simulink model "GIM81115_6_motor_model_prev_verision"  (R2024a)
settings: Solver=FixedStepAuto  StartTime=0.0  StopTime=inf  RelTol=1e-3
undefined symbols (not defined in the file): HS, IO291
libraries: speedgoatlib_IO691 x9, canmsglib x8, aru_toolbox x1, speedgoatlib_IO291 x1
settings Model: SimulationMode=external  ExtModeEnableFloating=off  Creator=claro  LastModifiedBy=user
settings SolverCC: ConcurrentTasks=on  PositivePriorityOrder=on
settings OptimizationCC: BlockReduction=off  OptimizeBlockIOStorage=off
settings DebuggingCC: TasksWithSamePriorityMsg=none
settings HardwareCC: ProdBitPerLong=64  ProdLongLongMode=on  ProdHWDeviceType=Intel->x86-64 (Linux 64)
settings RTWCC: Description=Speedgoat Real-Time Target Machine  SystemTargetFile=speedgoat.tlc  TemplateMakefile=slrealtime_default_tmf  Toolchain=Simulink Real-Time Toolchain  BuildConfiguration=Faster Runs  CodeExecutionProfiling=on  TargetLang=C++
settings SimulinkRealTimeTargetCC: InstructionSetFMA=off  LogToMDFFile=off

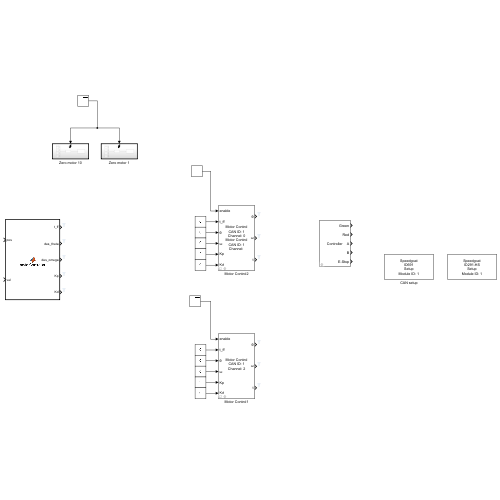
[thumbnail: Simulink's stored preview of the top-level diagram]
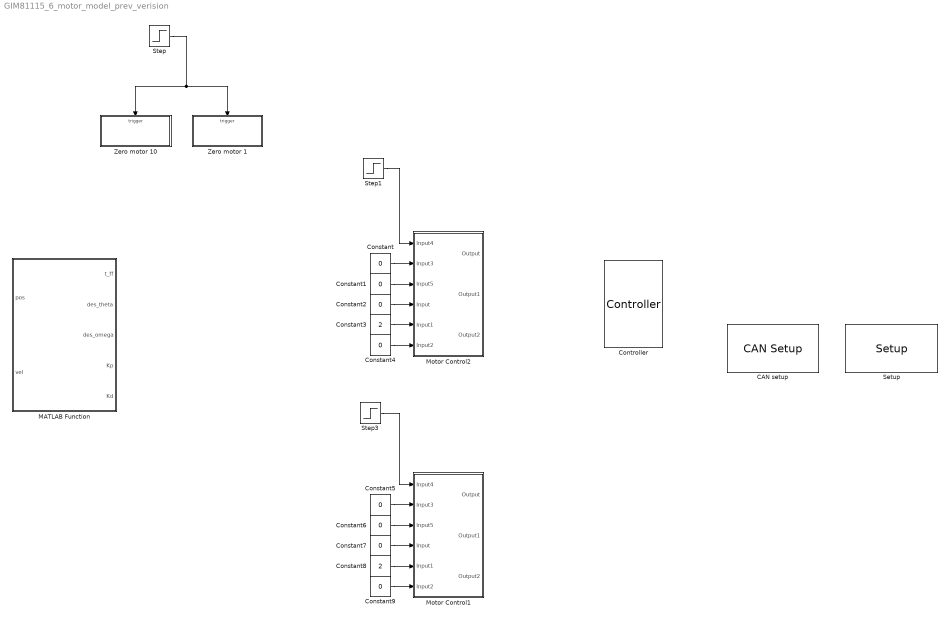
== system GIM81115_6_motor_model_prev_verision ==
  CAN setup : speedgoatlib_IO691/Legacy/CAN Setup   moduletype=IO691  id=1  pciSlot=-1  chn1=CAN (HS)  chn2=CAN (HS)  chn3=Disabled  chn4=Disabled  initStruct=[]  termStruct=[struct('Channel',1,'Protocol','CAN','BRS',0,'Type','Standard','Identifier',1,'Data',[255, 255, 255, 255, 255, 255, 255, 253],'Pause',0.001), struct('Channel',2,'Protocol','CAN','BRS',0,'Type','Standard','Identifier',2,'Data',[255, 255, 255, 255, 255, 255, 255, 253],'Pause',0.001)]  ArbitrationbdrChn1=1.0 MBaud  ArbitrationManbdrChn1=[2,8,31,8]  FdbdrChn1=1.0 MBaud  FdManbdrChn1=[2,8,31,8]  ArbitrationbdrChn2=1.0 MBaud  ArbitrationManbdrChn2=[2,8,31,8]  FdbdrChn2=1.0 MBaud  FdManbdrChn2=[2,8,31,8]  ArbitrationbdrChn3=1.0 MBaud  ArbitrationManbdrChn3=[2,8,31,8]  FdbdrChn3=5.0 MBaud  FdManbdrChn3=[2,2,5,2]  ArbitrationbdrChn4=1.0 MBaud  ArbitrationManbdrChn4=[2,8,31,8]  FdbdrChn4=5.0 MBaud  FdManbdrChn4=[2,2,5,2]  moduleInitValues=[691 1 -1 -1]
      settings: SourceProductName=IO691
  Constant{,1..2,4..7,9} (8 alike) : Constant  Value=0
  Constant3 : Constant  Value=2
  Constant8 : Constant  Value=2
  Controller : aru_toolbox/Controller
      settings: SourceProductName=ARU Toolbox
  MATLAB Function : MATLAB Function  TreatAsAtomicUnit=on
  Motor Control1 : Subsystem  AncestorBlock=aru_toolbox/Motor Control  mask(Motor Control){id=1, channel=2, offset=0}
      mask prompts: offset "Position Offset (rad)"
      mask help: Generic control block for motors running Ben Katz's motor control firmware. (https://github.com/bgkatz/motorcontrol)
      mask init:
      | % set_param([gcb '/write/CAN pack'],'MsgIdentifier',sprintf('%d',id));
      | set_param([gcb '/write/CAN Write Command'],'channel',sprintf('%d',channel));
      | set_param([gcb '/read/CAN Read State'],'channel',sprintf('%d',channel));
      | 
      | % set_param([gcb '/enable/CAN pack'],'MsgIdentifier',sprintf('%d',id));
      | set_param([gcb '/enable/CAN Write Motor Mode'],'channel',sprintf('%d',channel));
      | % motor termination message
      | % set_param([gcb '/CAN setup'],'termStruct',sprintf("[struct('Channel',%d,'Protocol','CAN','BRS',0,'Type','Standard','Identifier',%d,'Data',[255, 255, 255, 255, 255, 255, 255, 253],'Pause',0.001)]", channel, id))
      mask TypeOptions channel: 1 | 2
      mask DialogControl ParameterGroupVar Prompt: CAN
      mask DialogControl Container4 Prompt: Control
      mask Display:
      | fprintf('Motor Control\nCAN ID: %c\nChannel: %c\n', get_param(gcb,'id'), get_param(gcb,'channel'));
      | port_label('input',1,'enable');
      | port_label('input',2,'t_ff');
      | port_label('input',3,'θ');
      | port_label('input',4,'ω');
      | port_label('input',5,'Kp');
      | port_label('input',6,'Kd');
      | port_label('output',1,'θ');
      | port_label('output',2,'ω');
      | port_label('output',3,'t');
  Motor Control2 : Subsystem  AncestorBlock=aru_toolbox/Motor Control  mask(Motor Control){id=10, channel=1, offset=0}
      mask prompts: offset "Position Offset (rad)"
      mask help: Generic control block for motors running Ben Katz's motor control firmware. (https://github.com/bgkatz/motorcontrol)
      mask init: same as GIM81115_6_motor_model_prev_verision/Motor Control1
      mask TypeOptions channel: 1 | 2
      mask DialogControl ParameterGroupVar Prompt: CAN
      mask DialogControl Container4 Prompt: Control
      mask Display:
      | fprintf('Motor Control\nCAN ID: %c\nChannel: %c\n', get_param(gcb,'id'), get_param(gcb,'channel'));
      | port_label('input',1,'enable');
      | port_label('input',2,'t_ff');
      | port_label('input',3,'θ');
      | port_label('input',4,'ω');
      | port_label('input',5,'Kp');
      | port_label('input',6,'Kd');
      | port_label('output',1,'θ');
      | port_label('output',2,'ω');
      | port_label('output',3,'t');
  "Setup " : speedgoatlib_IO291/Setup   parInternalModuleId=1  parPciSlot=-1  parModuleId=1  parModuleType=IO291-HS  parTtlDoChannels=[]  parTtlDoInitValues=1  parTtlDoReset=1  parTtlDiChannels=[1 2 3 4 5]  parIsolDiChannels=[]  parFetDoChannels=[1 2 3 4 5 6]  parFetDoInitValues=0  parFetDoReset=1
      settings: SourceProductName=IO291
  Step : Step  Time=0.2  SampleTime=0
  Step1 : Step  SampleTime=0
  Step3 : Step  Time=2  SampleTime=0
  Zero motor 1 : Subsystem  TreatAsAtomicUnit=on
  Zero motor 10 : Subsystem  TreatAsAtomicUnit=on
  wires:
  Step/1 -> Zero motor 10/Trigger, Zero motor 1/Trigger
  Step1/1 -> Motor Control2/1(Input4)
  Constant/1 -> Motor Control2/2(Input3)
  Constant1/1 -> Motor Control2/3(Input5)
  Constant2/1 -> Motor Control2/4(Input)
  Constant3/1 -> Motor Control2/5(Input1)
  Constant4/1 -> Motor Control2/6(Input2)
  Constant9/1 -> Motor Control1/6(Input2)
  Constant6/1 -> Motor Control1/3(Input5)
  Step3/1 -> Motor Control1/1(Input4)
  Constant7/1 -> Motor Control1/4(Input)
  Constant5/1 -> Motor Control1/2(Input3)
  Constant8/1 -> Motor Control1/5(Input1)

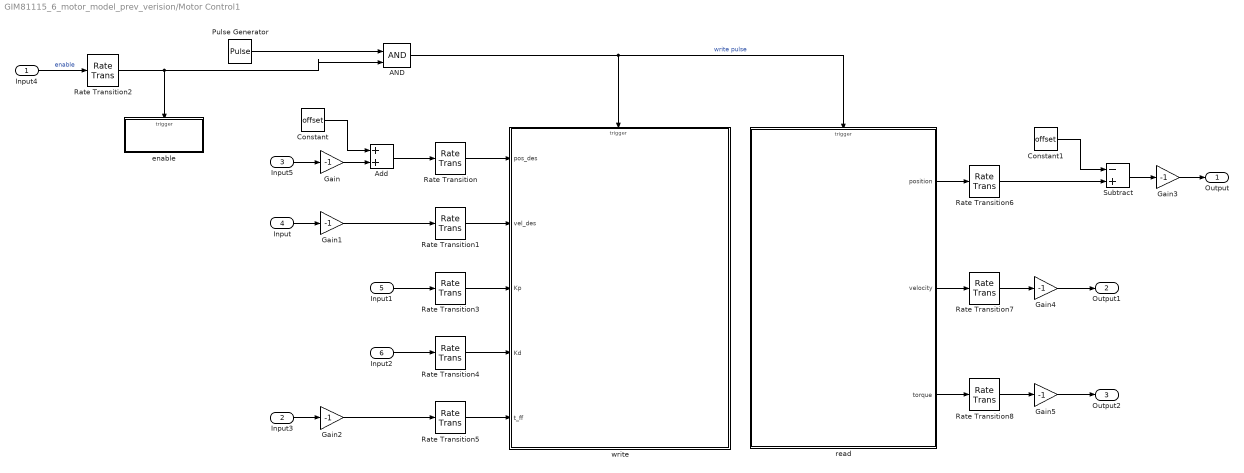
== system GIM81115_6_motor_model_prev_verision/Motor Control1 ==
  Input4 : Inport
  Input3 : Inport  Port=2
  Input5 : Inport  Port=3
  Input : Inport  Port=4
  Input1 : Inport  Port=5
  Input2 : Inport  Port=6
  AND : Logic  IconShape=distinctive  AllPortsSameDT=off  OutDataTypeStr=boolean
  Add : Sum
  Constant : Constant  Value=offset
  Constant1 : Constant  Value=offset
  Gain{,1..5} (6 alike) : Gain  Gain=-1
  Pulse Generator : DiscretePulseGenerator  PulseType=Time based  Period=0.001  PulseWidth=50
  Rate Transition{,1..8} (9 alike) : RateTransition
  Subtract : Sum  Inputs=-+
  enable : Subsystem  TreatAsAtomicUnit=on
  read : Subsystem  TreatAsAtomicUnit=on
  write : Subsystem  TreatAsAtomicUnit=on
  Output : Outport
  Output1 : Outport  Port=2
  Output2 : Outport  Port=3
  wires:
  Gain5/1 -> Output2/1
  Gain4/1 -> Output1/1
  Gain3/1 -> Output/1
  Gain2/1 -> Rate Transition5/1
  Gain1/1 -> Rate Transition1/1
  Gain/1 -> Add/2
  Constant1/1 -> Subtract/1
  Rate Transition6/1 -> Subtract/2
  Subtract/1 -> Gain3/1
  Constant/1 -> Add/1
  Add/1 -> Rate Transition/1
  Input5/1 -> Gain/1
  Rate Transition8/1 -> Gain5/1
  Rate Transition7/1 -> Gain4/1
  Rate Transition5/1 -> write/5(t_ff)
  Rate Transition4/1 -> write/4(Kd)
  Rate Transition3/1 -> write/3(Kp)
  Rate Transition2/1 -> enable/Trigger, AND/2
  Rate Transition1/1 -> write/2(vel_des)
  Rate Transition/1 -> write/1(pos_des)
  read/1(position) -> Rate Transition6/1
  Input4/1 -> Rate Transition2/1  "enable"
  AND/1 -> write/Trigger, read/Trigger  "write pulse"
  Pulse Generator/1 -> AND/1
  Input/1 -> Gain1/1
  read/3(torque) -> Rate Transition8/1
  read/2(velocity) -> Rate Transition7/1
  Input2/1 -> Rate Transition4/1
  Input3/1 -> Gain2/1
  Input1/1 -> Rate Transition3/1

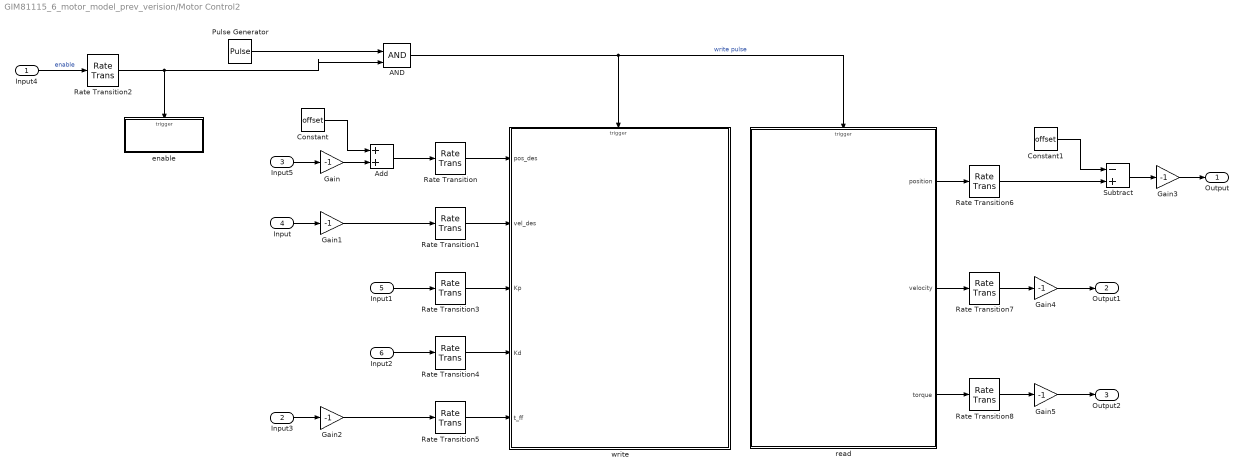
== system GIM81115_6_motor_model_prev_verision/Motor Control2 ==
  Input4 : Inport
  Input3 : Inport  Port=2
  Input5 : Inport  Port=3
  Input : Inport  Port=4
  Input1 : Inport  Port=5
  Input2 : Inport  Port=6
  AND : Logic  IconShape=distinctive  AllPortsSameDT=off  OutDataTypeStr=boolean
  Add : Sum
  Constant : Constant  Value=offset
  Constant1 : Constant  Value=offset
  Gain{,1..5} (6 alike) : Gain  Gain=-1
  Pulse Generator : DiscretePulseGenerator  PulseType=Time based  Period=0.001  PulseWidth=50
  Rate Transition{,1..8} (9 alike) : RateTransition
  Subtract : Sum  Inputs=-+
  enable : Subsystem  TreatAsAtomicUnit=on
  read : Subsystem  TreatAsAtomicUnit=on
  write : Subsystem  TreatAsAtomicUnit=on
  Output : Outport
  Output1 : Outport  Port=2
  Output2 : Outport  Port=3
  wires:
  Gain5/1 -> Output2/1
  Gain4/1 -> Output1/1
  Gain3/1 -> Output/1
  Gain2/1 -> Rate Transition5/1
  Gain1/1 -> Rate Transition1/1
  Gain/1 -> Add/2
  Constant1/1 -> Subtract/1
  Rate Transition6/1 -> Subtract/2
  Subtract/1 -> Gain3/1
  Constant/1 -> Add/1
  Add/1 -> Rate Transition/1
  Input5/1 -> Gain/1
  Rate Transition8/1 -> Gain5/1
  Rate Transition7/1 -> Gain4/1
  Rate Transition5/1 -> write/5(t_ff)
  Rate Transition4/1 -> write/4(Kd)
  Rate Transition3/1 -> write/3(Kp)
  Rate Transition2/1 -> enable/Trigger, AND/2
  Rate Transition1/1 -> write/2(vel_des)
  Rate Transition/1 -> write/1(pos_des)
  read/1(position) -> Rate Transition6/1
  Input4/1 -> Rate Transition2/1  "enable"
  AND/1 -> write/Trigger, read/Trigger  "write pulse"
  Pulse Generator/1 -> AND/1
  Input/1 -> Gain1/1
  read/3(torque) -> Rate Transition8/1
  read/2(velocity) -> Rate Transition7/1
  Input2/1 -> Rate Transition4/1
  Input3/1 -> Gain2/1
  Input1/1 -> Rate Transition3/1

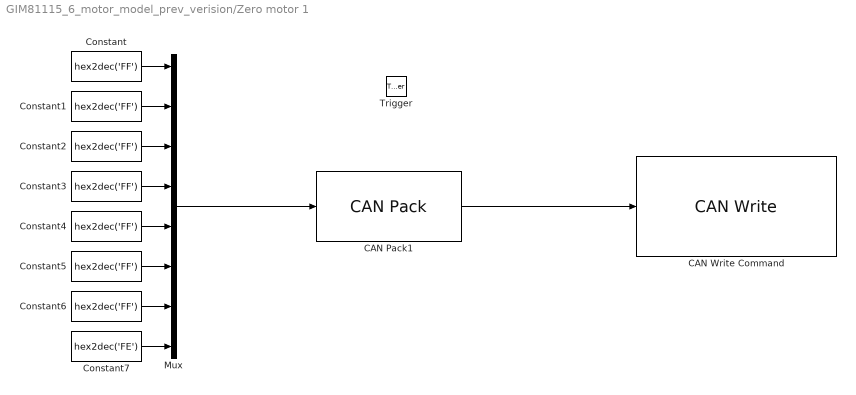
== system GIM81115_6_motor_model_prev_verision/Zero motor 1 ==
  Trigger : TriggerPort  VariantControl=Variant
  CAN Pack1 : canmsglib/CAN Pack  MsgList=(none)  MsgName=CAN Msg  MsgIDType=Standard (11-bit identifier)  MsgIdentifier=1  MsgLength=8  Remote=off  ApplyMinMax=off  BusOutput=off  SignalInfo={}
      settings: DataFormat=raw data
  CAN Write Command : speedgoatlib_IO691/Legacy/CAN Write  id=1  ts=-1  channel=2  messageType=CAN  BusInput=off  enableStatusPort=off  canType=CAN (HS)  initValues=[691 1 -1 1 1 1 0 0]
      settings: SourceProductName=IO691
  Constant{,1..6} (7 alike) : Constant  Value=hex2dec('FF')  OutDataTypeStr=uint8  SampleTime=-1
  Constant7 : Constant  Value=hex2dec('FE')  OutDataTypeStr=uint8  SampleTime=-1
  Mux : Mux  Inputs=8
  wires:
  Constant1/1 -> Mux/2
  Mux/1 -> CAN Pack1/1
  Constant/1 -> Mux/1
  Constant6/1 -> Mux/7
  Constant4/1 -> Mux/5
  Constant7/1 -> Mux/8
  Constant3/1 -> Mux/4
  Constant5/1 -> Mux/6
  Constant2/1 -> Mux/3
  CAN Pack1/1 -> CAN Write Command/1

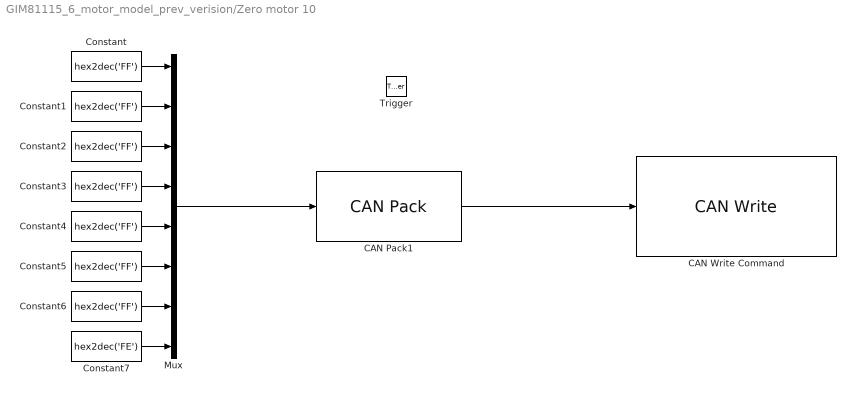
== system GIM81115_6_motor_model_prev_verision/Zero motor 10 ==
  Trigger : TriggerPort  VariantControl=Variant
  CAN Pack1 : canmsglib/CAN Pack  MsgList=(none)  MsgName=CAN Msg  MsgIDType=Standard (11-bit identifier)  MsgIdentifier=10  MsgLength=8  Remote=off  ApplyMinMax=off  BusOutput=off  SignalInfo={}
      settings: DataFormat=raw data
  CAN Write Command : speedgoatlib_IO691/Legacy/CAN Write  id=1  ts=-1  channel=1  messageType=CAN  BusInput=off  enableStatusPort=off  canType=CAN (HS)  initValues=[691 1 -1 0 1 1 0 0]
      settings: SourceProductName=IO691
  Constant{,1..6} (7 alike) : Constant  Value=hex2dec('FF')  OutDataTypeStr=uint8  SampleTime=-1
  Constant7 : Constant  Value=hex2dec('FE')  OutDataTypeStr=uint8  SampleTime=-1
  Mux : Mux  Inputs=8
  wires:
  Constant1/1 -> Mux/2
  Mux/1 -> CAN Pack1/1
  Constant/1 -> Mux/1
  Constant6/1 -> Mux/7
  Constant4/1 -> Mux/5
  Constant7/1 -> Mux/8
  Constant3/1 -> Mux/4
  Constant5/1 -> Mux/6
  Constant2/1 -> Mux/3
  CAN Pack1/1 -> CAN Write Command/1

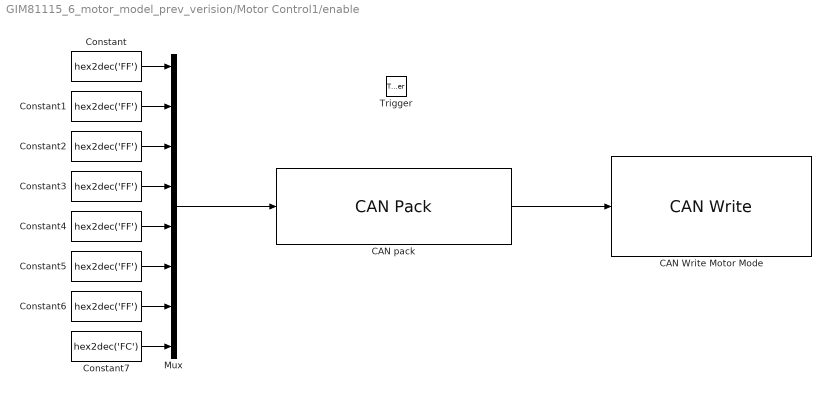
== system GIM81115_6_motor_model_prev_verision/Motor Control1/enable ==
  Trigger : TriggerPort  VariantControl=Variant
  CAN Write Motor Mode : speedgoatlib_IO691/Legacy/CAN Write  id=1  ts=-1  channel=2  messageType=CAN  BusInput=off  enableStatusPort=off  canType=CAN (HS)  initValues=[691 1 -1 1 1 1 0 0]
      settings: SourceProductName=IO691
  CAN pack : canmsglib/CAN Pack  MsgList=(none)  MsgName=enable  MsgIDType=Standard (11-bit identifier)  MsgIdentifier=id  MsgLength=8  Remote=off  ApplyMinMax=off  BusOutput=off  SignalInfo={ 'Motor postition 8-H', '0', '8', 'LE', 'unsigned', 'Standard', '0', '1', '0', '-Inf', 'Inf'; 'Motor position 8-L', '8', '8', 'LE', 'unsigned', 'Standard', '0', '1', '0', '-Inf', 'Inf'; 'Motor seed 8-H', '16', '8', 'LE', 'unsigned', 'Standard', '0', '1', '0', '-Inf', 'Inf'; 'Motor speed 4-L', '28', '4', 'LE', 'unsigned', 'Standard', '0', '1', '0', '-Inf', 'Inf'; 'KP 4-H', '24', '4', 'LE', 'unsigned', 'Standard', '0', '1', '0', '-Inf', 'Inf'; 'KP 8-L', '32', '8', 'LE', 'unsigned', 'Standard', '0', '1', '0', '-Inf', 'Inf'; 'KP 8-H', '40', '8', 'LE', 'unsigned', 'Standard', '0', '1', '0', '-Inf', 'Inf'; 'KD 4-L', '52', '4', 'LE', 'unsigned', 'Standard', '0', '1', '0', '-Inf', 'Inf'; 'Current 4-H', '48', '4', 'LE', 'unsigned', 'Standard', '0', '1', '0', '-Inf', 'Inf'; 'Current 8-L', '56', '8', 'LE', 'unsigned', 'Standard', '0', '1', '0', '-Inf', 'Inf' }
      settings: DataFormat=raw data
  Constant{,1..6} (7 alike) : Constant  Value=hex2dec('FF')  OutDataTypeStr=uint8  SampleTime=-1
  Constant7 : Constant  Value=hex2dec('FC')  OutDataTypeStr=uint8  SampleTime=-1
  Mux : Mux  Inputs=8
  wires:
  Constant6/1 -> Mux/7
  Constant/1 -> Mux/1
  Constant2/1 -> Mux/3
  Constant3/1 -> Mux/4
  Constant5/1 -> Mux/6
  Constant1/1 -> Mux/2
  Constant4/1 -> Mux/5
  Constant7/1 -> Mux/8
  Mux/1 -> CAN pack/1
  CAN pack/1 -> CAN Write Motor Mode/1

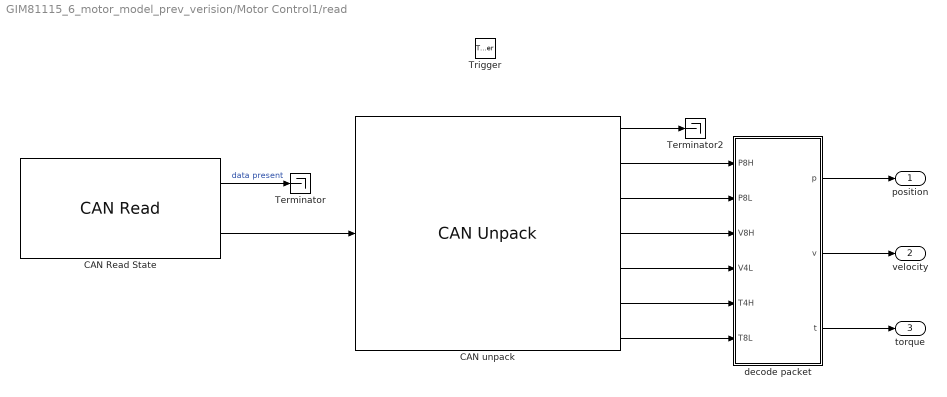
== system GIM81115_6_motor_model_prev_verision/Motor Control1/read ==
  Trigger : TriggerPort  TriggerType=either  VariantControl=Variant
  CAN Read State : speedgoatlib_IO691/Legacy/CAN Read  id=1  ts=-1  channel=2  messageType=CAN  canType=CAN (HS)  BusOutput=off  initValues=[691 1 -1 1 1 1 0]
      settings: SourceProductName=IO691
  CAN unpack : canmsglib/CAN Unpack  MsgList=(none)  MsgName=CAN Msg  MsgIDType=Standard (11-bit identifier)  MsgIdentifier=0  MsgLength=6  SignalInfo={ 'ID', '0', '8', 'LE', 'unsigned', 'Standard', '0', '1', '0', '-Inf', 'Inf'; 'P8H', '8', '8', 'LE', 'unsigned', 'Standard', '0', '1', '0', '-Inf', 'Inf'; 'P8L', '16', '8', 'LE', 'unsigned', 'Standard', '0', '1', '0', '-Inf', 'Inf'; 'V8H', '24', '8', 'LE', 'unsigned', 'Standard', '0', '1', '0', '-Inf', 'Inf'; 'V4L', '36', '4', 'LE', 'unsigned', 'Standard', '0', '1', '0', '-Inf', 'Inf'; 'I4H', '32', '4', 'LE', 'unsigned', 'Standard', '0', '1', '0', '-Inf', 'Inf'; 'I8L', '40', '8', 'LE', 'unsigned', 'Standard', '0', '1', '0', '-Inf', 'Inf' }  IDPort=off  TimestampPort=off  ErrorPort=off  RemotePort=off  LengthPort=off  StatusPort=off  ApplyMinMax=off
  Terminator : Terminator
  Terminator2 : Terminator
  decode packet : MATLAB Function  TreatAsAtomicUnit=on
  position : Outport
  velocity : Outport  Port=2
  torque : Outport  Port=3
  wires:
  CAN Read State/1 -> Terminator/1  "data present"
  decode packet/3(t) -> torque/1
  decode packet/1(p) -> position/1
  decode packet/2(v) -> velocity/1
  CAN unpack/4 -> decode packet/3(V8H)
  CAN unpack/7 -> decode packet/6(T8L)
  CAN unpack/2 -> decode packet/1(P8H)
  CAN unpack/3 -> decode packet/2(P8L)
  CAN unpack/5 -> decode packet/4(V4L)
  CAN unpack/6 -> decode packet/5(T4H)
  CAN Read State/2 -> CAN unpack/1
  CAN unpack/1 -> Terminator2/1

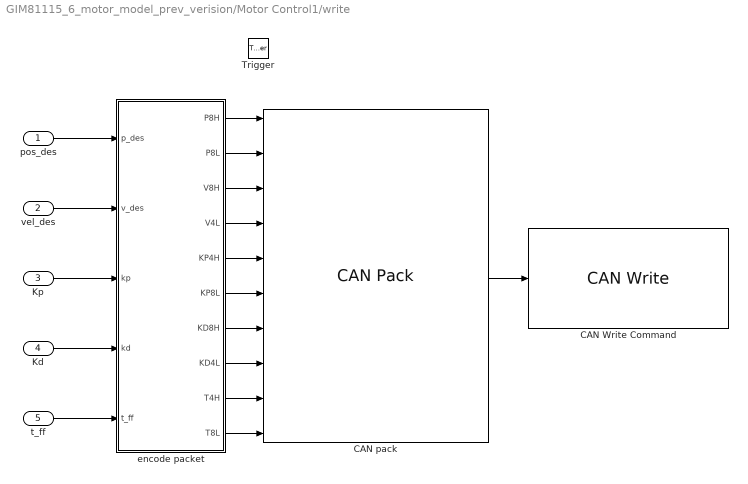
== system GIM81115_6_motor_model_prev_verision/Motor Control1/write ==
  pos_des : Inport
  vel_des : Inport  Port=2
  Kp : Inport  Port=3
  Kd : Inport  Port=4
  t_ff : Inport  Port=5
  Trigger : TriggerPort  VariantControl=Variant
  CAN Write Command : speedgoatlib_IO691/Legacy/CAN Write  id=1  ts=-1  channel=2  messageType=CAN  BusInput=off  enableStatusPort=off  canType=CAN (HS)  initValues=[691 1 -1 1 1 1 0 0]
      settings: SourceProductName=IO691
  CAN pack : canmsglib/CAN Pack  MsgList=(none)  MsgName=MotorControl  MsgIDType=Standard (11-bit identifier)  MsgIdentifier=id  MsgLength=8  Remote=off  ApplyMinMax=off  BusOutput=off  SignalInfo={ 'P8H', '0', '8', 'LE', 'unsigned', 'Standard', '0', '1', '0', '-Inf', 'Inf'; 'P8L', '8', '8', 'LE', 'unsigned', 'Standard', '0', '1', '0', '-Inf', 'Inf'; 'V8H', '16', '8', 'LE', 'unsigned', 'Standard', '0', '1', '0', '-Inf', 'Inf'; 'V4L', '28', '4', 'LE', 'unsigned', 'Standard', '0', '1', '0', '-Inf', 'Inf'; 'KP4H', '24', '4', 'LE', 'unsigned', 'Standard', '0', '1', '0', '-Inf', 'Inf'; 'KP8L', '32', '8', 'LE', 'unsigned', 'Standard', '0', '1', '0', '-Inf', 'Inf'; 'KD8H', '40', '8', 'LE', 'unsigned', 'Standard', '0', '1', '0', '-Inf', 'Inf'; 'KD4L', '52', '4', 'LE', 'unsigned', 'Standard', '0', '1', '0', '-Inf', 'Inf'; 'T4H', '48', '4', 'LE', 'unsigned', 'Standard', '0', '1', '0', '-Inf', 'Inf'; 'T8L', '56', '8', 'LE', 'unsigned', 'Standard', '0', '1', '0', '-Inf', 'Inf' }
      settings: DataFormat=manually specified signals
  encode packet : MATLAB Function  TreatAsAtomicUnit=on
  wires:
  encode packet/10(T8L) -> CAN pack/10
  encode packet/3(V8H) -> CAN pack/3
  CAN pack/1 -> CAN Write Command/1
  encode packet/1(P8H) -> CAN pack/1
  encode packet/9(T4H) -> CAN pack/9
  encode packet/4(V4L) -> CAN pack/4
  encode packet/8(KD4L) -> CAN pack/8
  t_ff/1 -> encode packet/5(t_ff)
  Kd/1 -> encode packet/4(kd)
  encode packet/5(KP4H) -> CAN pack/5
  Kp/1 -> encode packet/3(kp)
  encode packet/2(P8L) -> CAN pack/2
  encode packet/7(KD8H) -> CAN pack/7
  encode packet/6(KP8L) -> CAN pack/6
  pos_des/1 -> encode packet/1(p_des)
  vel_des/1 -> encode packet/2(v_des)

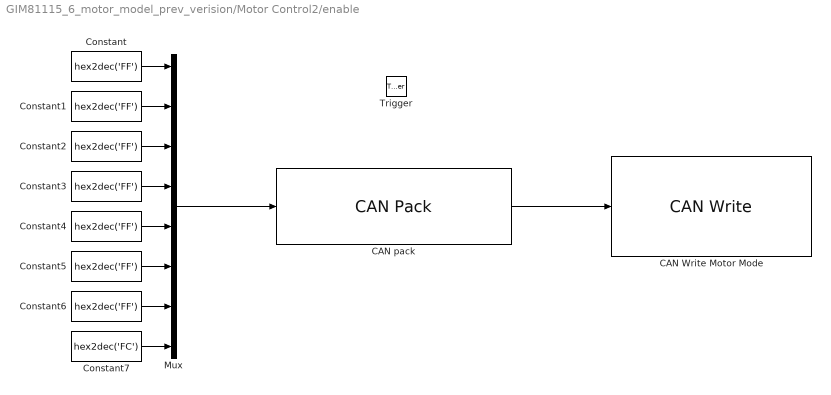
== system GIM81115_6_motor_model_prev_verision/Motor Control2/enable ==
  Trigger : TriggerPort  VariantControl=Variant
  CAN Write Motor Mode : speedgoatlib_IO691/Legacy/CAN Write  id=1  ts=-1  channel=1  messageType=CAN  BusInput=off  enableStatusPort=off  canType=CAN (HS)  initValues=[691 1 -1 0 1 1 0 0]
      settings: SourceProductName=IO691
  CAN pack : canmsglib/CAN Pack  MsgList=(none)  MsgName=enable  MsgIDType=Standard (11-bit identifier)  MsgIdentifier=id  MsgLength=8  Remote=off  ApplyMinMax=off  BusOutput=off  SignalInfo={ 'Motor postition 8-H', '0', '8', 'LE', 'unsigned', 'Standard', '0', '1', '0', '-Inf', 'Inf'; 'Motor position 8-L', '8', '8', 'LE', 'unsigned', 'Standard', '0', '1', '0', '-Inf', 'Inf'; 'Motor seed 8-H', '16', '8', 'LE', 'unsigned', 'Standard', '0', '1', '0', '-Inf', 'Inf'; 'Motor speed 4-L', '28', '4', 'LE', 'unsigned', 'Standard', '0', '1', '0', '-Inf', 'Inf'; 'KP 4-H', '24', '4', 'LE', 'unsigned', 'Standard', '0', '1', '0', '-Inf', 'Inf'; 'KP 8-L', '32', '8', 'LE', 'unsigned', 'Standard', '0', '1', '0', '-Inf', 'Inf'; 'KP 8-H', '40', '8', 'LE', 'unsigned', 'Standard', '0', '1', '0', '-Inf', 'Inf'; 'KD 4-L', '52', '4', 'LE', 'unsigned', 'Standard', '0', '1', '0', '-Inf', 'Inf'; 'Current 4-H', '48', '4', 'LE', 'unsigned', 'Standard', '0', '1', '0', '-Inf', 'Inf'; 'Current 8-L', '56', '8', 'LE', 'unsigned', 'Standard', '0', '1', '0', '-Inf', 'Inf' }
      settings: DataFormat=raw data
  Constant{,1..6} (7 alike) : Constant  Value=hex2dec('FF')  OutDataTypeStr=uint8  SampleTime=-1
  Constant7 : Constant  Value=hex2dec('FC')  OutDataTypeStr=uint8  SampleTime=-1
  Mux : Mux  Inputs=8
  wires:
  Constant6/1 -> Mux/7
  Constant/1 -> Mux/1
  Constant2/1 -> Mux/3
  Constant3/1 -> Mux/4
  Constant5/1 -> Mux/6
  Constant1/1 -> Mux/2
  Constant4/1 -> Mux/5
  Constant7/1 -> Mux/8
  Mux/1 -> CAN pack/1
  CAN pack/1 -> CAN Write Motor Mode/1

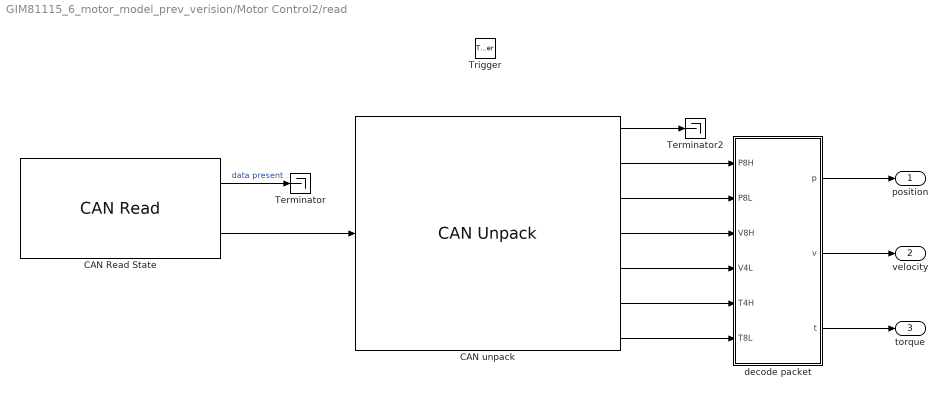
== system GIM81115_6_motor_model_prev_verision/Motor Control2/read ==
  Trigger : TriggerPort  TriggerType=either  VariantControl=Variant
  CAN Read State : speedgoatlib_IO691/Legacy/CAN Read  id=1  ts=-1  channel=1  messageType=CAN  canType=CAN (HS)  BusOutput=off  initValues=[691 1 -1 0 1 1 0]
      settings: SourceProductName=IO691
  CAN unpack : canmsglib/CAN Unpack  MsgList=(none)  MsgName=CAN Msg  MsgIDType=Standard (11-bit identifier)  MsgIdentifier=0  MsgLength=6  SignalInfo={ 'ID', '0', '8', 'LE', 'unsigned', 'Standard', '0', '1', '0', '-Inf', 'Inf'; 'P8H', '8', '8', 'LE', 'unsigned', 'Standard', '0', '1', '0', '-Inf', 'Inf'; 'P8L', '16', '8', 'LE', 'unsigned', 'Standard', '0', '1', '0', '-Inf', 'Inf'; 'V8H', '24', '8', 'LE', 'unsigned', 'Standard', '0', '1', '0', '-Inf', 'Inf'; 'V4L', '36', '4', 'LE', 'unsigned', 'Standard', '0', '1', '0', '-Inf', 'Inf'; 'I4H', '32', '4', 'LE', 'unsigned', 'Standard', '0', '1', '0', '-Inf', 'Inf'; 'I8L', '40', '8', 'LE', 'unsigned', 'Standard', '0', '1', '0', '-Inf', 'Inf' }  IDPort=off  TimestampPort=off  ErrorPort=off  RemotePort=off  LengthPort=off  StatusPort=off  ApplyMinMax=off
  Terminator : Terminator
  Terminator2 : Terminator
  decode packet : MATLAB Function  TreatAsAtomicUnit=on
  position : Outport
  velocity : Outport  Port=2
  torque : Outport  Port=3
  wires:
  CAN Read State/1 -> Terminator/1  "data present"
  decode packet/3(t) -> torque/1
  decode packet/1(p) -> position/1
  decode packet/2(v) -> velocity/1
  CAN unpack/4 -> decode packet/3(V8H)
  CAN unpack/7 -> decode packet/6(T8L)
  CAN unpack/2 -> decode packet/1(P8H)
  CAN unpack/3 -> decode packet/2(P8L)
  CAN unpack/5 -> decode packet/4(V4L)
  CAN unpack/6 -> decode packet/5(T4H)
  CAN Read State/2 -> CAN unpack/1
  CAN unpack/1 -> Terminator2/1

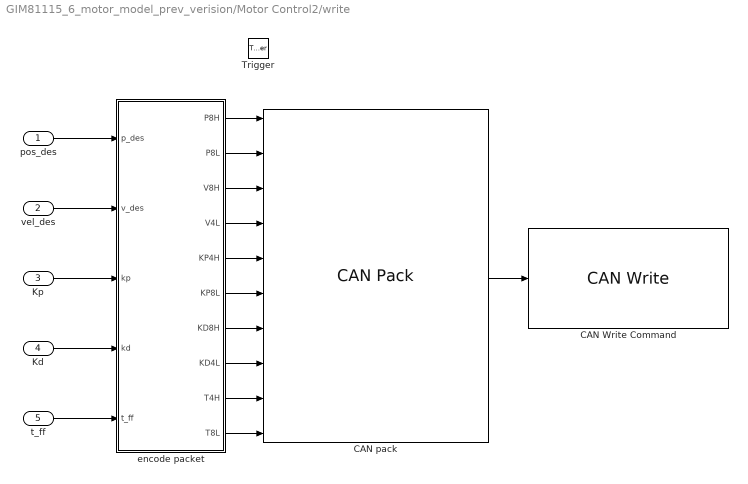
== system GIM81115_6_motor_model_prev_verision/Motor Control2/write ==
  pos_des : Inport
  vel_des : Inport  Port=2
  Kp : Inport  Port=3
  Kd : Inport  Port=4
  t_ff : Inport  Port=5
  Trigger : TriggerPort  VariantControl=Variant
  CAN Write Command : speedgoatlib_IO691/Legacy/CAN Write  id=1  ts=-1  channel=1  messageType=CAN  BusInput=off  enableStatusPort=off  canType=CAN (HS)  initValues=[691 1 -1 0 1 1 0 0]
      settings: SourceProductName=IO691
  CAN pack : canmsglib/CAN Pack  MsgList=(none)  MsgName=MotorControl  MsgIDType=Standard (11-bit identifier)  MsgIdentifier=id  MsgLength=8  Remote=off  ApplyMinMax=off  BusOutput=off  SignalInfo={ 'P8H', '0', '8', 'LE', 'unsigned', 'Standard', '0', '1', '0', '-Inf', 'Inf'; 'P8L', '8', '8', 'LE', 'unsigned', 'Standard', '0', '1', '0', '-Inf', 'Inf'; 'V8H', '16', '8', 'LE', 'unsigned', 'Standard', '0', '1', '0', '-Inf', 'Inf'; 'V4L', '28', '4', 'LE', 'unsigned', 'Standard', '0', '1', '0', '-Inf', 'Inf'; 'KP4H', '24', '4', 'LE', 'unsigned', 'Standard', '0', '1', '0', '-Inf', 'Inf'; 'KP8L', '32', '8', 'LE', 'unsigned', 'Standard', '0', '1', '0', '-Inf', 'Inf'; 'KD8H', '40', '8', 'LE', 'unsigned', 'Standard', '0', '1', '0', '-Inf', 'Inf'; 'KD4L', '52', '4', 'LE', 'unsigned', 'Standard', '0', '1', '0', '-Inf', 'Inf'; 'T4H', '48', '4', 'LE', 'unsigned', 'Standard', '0', '1', '0', '-Inf', 'Inf'; 'T8L', '56', '8', 'LE', 'unsigned', 'Standard', '0', '1', '0', '-Inf', 'Inf' }
      settings: DataFormat=manually specified signals
  encode packet : MATLAB Function  TreatAsAtomicUnit=on
  wires:
  encode packet/10(T8L) -> CAN pack/10
  encode packet/3(V8H) -> CAN pack/3
  CAN pack/1 -> CAN Write Command/1
  encode packet/1(P8H) -> CAN pack/1
  encode packet/9(T4H) -> CAN pack/9
  encode packet/4(V4L) -> CAN pack/4
  encode packet/8(KD4L) -> CAN pack/8
  t_ff/1 -> encode packet/5(t_ff)
  Kd/1 -> encode packet/4(kd)
  encode packet/5(KP4H) -> CAN pack/5
  Kp/1 -> encode packet/3(kp)
  encode packet/2(P8L) -> CAN pack/2
  encode packet/7(KD8H) -> CAN pack/7
  encode packet/6(KP8L) -> CAN pack/6
  pos_des/1 -> encode packet/1(p_des)
  vel_des/1 -> encode packet/2(v_des)

== matlab function GIM81115_6_motor_model_prev_verision/Motor Control1/read/decode packet ==
  data: P8H input; p output; P8L input; V8H input; V4L input; T4H input; T8L input; v output; t output
function [p, v, t] = decode(P8H,P8L,V8H,V4L,T4H,T8L)
    % MOTOR CONSTANTS
    GR = 6; % Gear ratio
    KT = 0.28; % Torque Constant Nm/A
    P_MAX = 12.5; % rad
    P_MIN = -P_MAX; % rad
    V_MAX = 65.0; % rad/s
    V_MIN = -V_MAX; % rad/s
    I_MAX = 20.0; % A
    T_MAX = I_MAX*KT*GR; % Nm
    T_MIN = -I_MAX*KT*GR; % Nm
    KP_MAX = 500; % Nm/rad
    KP_MIN = 0; % Nm/rad
    KD_MAX = 5; % Nm/rad/s
    KD_MIN = 0; % Nm/rad/s    

    % combine data
    p_int = bitor(bitshift(P8H, 8), P8L);
    v_int = bitor(bitshift(V8H, 4), V4L);
    t_int = bitor(bitshift(T4H, 8), T8L);
    
    % convert uints to floats
    p = uint_to_float(p_int, P_MIN, P_MAX, 16);
    v = uint_to_float(v_int, V_MIN, V_MAX, 12);
    t = uint_to_float(t_int, T_MIN, T_MAX, 12);

    % Converts a float to an unsigned int, given range and number of bits
    function x_float = uint_to_float(x, x_min, x_max, n_bits)
        span = x_max - x_min;
        offset = x_min;
        x_float = x * span / (bitshift(1, n_bits)-1) + offset;
    end
end

== matlab function GIM81115_6_motor_model_prev_verision/MATLAB Function ==
  data: t_ff output; des_theta output; des_omega output; pos input; vel input; Kp output; Kd output
function [t_ff, des_theta, des_omega, Kp, Kd] = motorController(pos, vel)

    % Params
    J =  0.000072; % [kg*m^2]
    Kt = 1.84; % Torque Constant [Nm/A]
    I_max = 4.8; % Max Current [A]
    T_s = 0.05; % Settling time [s]
    zeta = 0.7; % Damping Ratio -> Underdamped
    t_limit = 1; % Torque Limit
    
    % Calculate Maximum Torque
    T_max = Kt * I_max;
    
    % Calcualte natural frequency
    wn = 4 / (zeta * T_s);
    
    if (pos <  -90 *pi/180) % Apply electrical break if close to mechanical limits
        des_theta = -85*pi/180;
        des_omega = 0;
        stop_distance = 5*pi/180;
        Kp = T_max/stop_distance;
        Kd = 2 * sqrt(J * Kp);
        t_ff = 0;
    elseif (pos > 90*pi/180)
        des_theta = 85*pi/180;
        des_omega = 0;
        stop_distance = 5*pi/180;
        Kp = T_max/stop_distance;
        Kd = 2 * sqrt(J * Kp);
        t_ff = 0;
    else
        des_theta = 0;
        des_omega = 0;
        Kp = J * wn^2;
        Kd = 2 * zeta * sqrt(J * Kp);
        t_ff = 0;
    end

    % Calculate comanded toruqe
    t_cmd = Kp* (des_theta - pos) + Kd * (des_omega - vel);
    t_tot = t_cmd + t_ff;

    % Scale gains 
    if abs(t_tot) > t_limit
        scale_factor = abs (t_limit/ t_tot);
        Kp = Kp * scale_factor;
        Kd = Kd * scale_factor;
    end

end

== matlab function GIM81115_6_motor_model_prev_verision/Motor Control1/write/encode packet ==
  data: p_des input; P8H output; v_des input; kp input; kd input; t_ff input; P8L output; V8H output; V4L output; KP4H output; KP8L output; KD8H output; KD4L output; T4H output; T8L output
function [P8H,P8L,V8H,V4L,KP4H,KP8L,KD8H,KD4L,T4H,T8L] = encode(p_des, v_des, kp, kd, t_ff)
    % MOTOR CONSTANTS
    GR = 6; % Gear ratio
    KT = 0.28; % Torque Constant Nm/A
    P_MAX = 12.5; % rad
    P_MIN = -P_MAX; % rad
    V_MAX = 65.0; % rad/s
    V_MIN = -V_MAX; % rad/s
    I_MAX = 20.0; % A
    T_MAX = I_MAX*KT*GR; % Nm
    T_MIN = -I_MAX*KT*GR; % Nm
    KP_MAX = 500; % Nm/rad
    KP_MIN = 0; % Nm/rad
    KD_MAX = 5; % Nm/rad/s
    KD_MIN = 0; % Nm/rad/s
    % bound inputs
    p_des = min([max([P_MIN,p_des]),P_MAX]);
    v_des = min([max([V_MIN,v_des]),V_MAX]);
    kp = min([max([KP_MIN,kp]),KP_MAX]);
    kd = min([max([KD_MIN,kd]),KD_MAX]);
    t_ff = min([max([T_MIN,t_ff]),T_MAX]);
    
    % convert floats to unsigned integers
    p_int = float_to_uint(p_des, P_MIN, P_MAX, 16);
    v_int = float_to_uint(v_des, V_MIN, V_MAX, 12);
    kp_int = float_to_uint(kp, KP_MIN, KP_MAX, 12);
    kd_int = float_to_uint(kd, KD_MIN, KD_MAX, 12);
    t_int = float_to_uint(t_ff, T_MIN, T_MAX, 12);
    
    % break up for CAN frame 
    P8H = bitshift(p_int, -8); % 8 higher bits
    P8L = bitand(p_int, 0xFF); % 8 lower bits
    V8H = bitshift(v_int, -4); % 8 higher bits
    V4L = bitand(v_int, 0xF); % 4 lower bits
    KP4H = bitshift(kp_int, -8); % 4 higher bits
    KP8L = bitand(kp_int, 0xFF); % 8 lower bits
    KD8H = bitshift(kd_int, -4); % 8 higher bits
    KD4L = bitand(kd_int, 0xF); % 4 lower bits
    T4H = bitshift(t_int, -8); % 4 higher bits
    T8L = bitand(t_int, 0xFF); % 8 lower bits
    
    % Converts a float to an unsigned int, given range and number of bits
    function x_int = float_to_uint(x, x_min, x_max, n_bits)
        span = x_max - x_min;
        min([max([x_min,x]),x_max])
        x_int = ((x - x_min)*(bitshift(1, n_bits) / span));
    end
end
%final_values = desired_pos,desired_vel,desired_kp,desired_kd,desired_tau;

== matlab function GIM81115_6_motor_model_prev_verision/Motor Control2/read/decode packet ==
  data: P8H input; p output; P8L input; V8H input; V4L input; T4H input; T8L input; v output; t output
function [p, v, t] = decode(P8H,P8L,V8H,V4L,T4H,T8L)
    % MOTOR CONSTANTS
    GR = 6; % Gear ratio
    KT = 0.28; % Torque Constant Nm/A
    P_MAX = 12.5; % rad
    P_MIN = -P_MAX; % rad
    V_MAX = 65.0; % rad/s
    V_MIN = -V_MAX; % rad/s
    I_MAX = 20.0; % A
    T_MAX = I_MAX*KT*GR; % Nm
    T_MIN = -I_MAX*KT*GR; % Nm
    KP_MAX = 500; % Nm/rad
    KP_MIN = 0; % Nm/rad
    KD_MAX = 5; % Nm/rad/s
    KD_MIN = 0; % Nm/rad/s    

    % combine data
    p_int = bitor(bitshift(P8H, 8), P8L);
    v_int = bitor(bitshift(V8H, 4), V4L);
    t_int = bitor(bitshift(T4H, 8), T8L);
    
    % convert uints to floats
    p = uint_to_float(p_int, P_MIN, P_MAX, 16);
    v = uint_to_float(v_int, V_MIN, V_MAX, 12);
    t = uint_to_float(t_int, T_MIN, T_MAX, 12);

    % Converts a float to an unsigned int, given range and number of bits
    function x_float = uint_to_float(x, x_min, x_max, n_bits)
        span = x_max - x_min;
        offset = x_min;
        x_float = x * span / (bitshift(1, n_bits)-1) + offset;
    end
end

== matlab function GIM81115_6_motor_model_prev_verision/Motor Control2/write/encode packet ==
  data: p_des input; P8H output; v_des input; kp input; kd input; t_ff input; P8L output; V8H output; V4L output; KP4H output; KP8L output; KD8H output; KD4L output; T4H output; T8L output
function [P8H,P8L,V8H,V4L,KP4H,KP8L,KD8H,KD4L,T4H,T8L] = encode(p_des, v_des, kp, kd, t_ff)
    % MOTOR CONSTANTS
    GR = 6; % Gear ratio
    KT = 0.28; % Torque Constant Nm/A
    P_MAX = 12.5; % rad
    P_MIN = -P_MAX; % rad
    V_MAX = 65.0; % rad/s
    V_MIN = -V_MAX; % rad/s
    I_MAX = 20.0; % A
    T_MAX = I_MAX*KT*GR; % Nm
    T_MIN = -I_MAX*KT*GR; % Nm
    KP_MAX = 500; % Nm/rad
    KP_MIN = 0; % Nm/rad
    KD_MAX = 5; % Nm/rad/s
    KD_MIN = 0; % Nm/rad/s
    % bound inputs
    p_des = min([max([P_MIN,p_des]),P_MAX]);
    v_des = min([max([V_MIN,v_des]),V_MAX]);
    kp = min([max([KP_MIN,kp]),KP_MAX]);
    kd = min([max([KD_MIN,kd]),KD_MAX]);
    t_ff = min([max([T_MIN,t_ff]),T_MAX]);
    
    % convert floats to unsigned integers
    p_int = float_to_uint(p_des, P_MIN, P_MAX, 16);
    v_int = float_to_uint(v_des, V_MIN, V_MAX, 12);
    kp_int = float_to_uint(kp, KP_MIN, KP_MAX, 12);
    kd_int = float_to_uint(kd, KD_MIN, KD_MAX, 12);
    t_int = float_to_uint(t_ff, T_MIN, T_MAX, 12);
    
    % break up for CAN frame 
    P8H = bitshift(p_int, -8); % 8 higher bits
    P8L = bitand(p_int, 0xFF); % 8 lower bits
    V8H = bitshift(v_int, -4); % 8 higher bits
    V4L = bitand(v_int, 0xF); % 4 lower bits
    KP4H = bitshift(kp_int, -8); % 4 higher bits
    KP8L = bitand(kp_int, 0xFF); % 8 lower bits
    KD8H = bitshift(kd_int, -4); % 8 higher bits
    KD4L = bitand(kd_int, 0xF); % 4 lower bits
    T4H = bitshift(t_int, -8); % 4 higher bits
    T8L = bitand(t_int, 0xFF); % 8 lower bits
    
    % Converts a float to an unsigned int, given range and number of bits
    function x_int = float_to_uint(x, x_min, x_max, n_bits)
        span = x_max - x_min;
        min([max([x_min,x]),x_max])
        x_int = ((x - x_min)*(bitshift(1, n_bits) / span));
    end
end
%final_values = desired_pos,desired_vel,desired_kp,desired_kd,desired_tau;
